simulink model "testmpc"  (R2021a)
settings: Solver=VariableStepAuto  StartTime=0.0  StopTime=10.0  RelTol=1e-3
undefined symbols (not defined in the file or in its folder): sigbuilder_block
libraries: mpclib x1
settings Model: Creator=uddin  LastModifiedBy=uddin

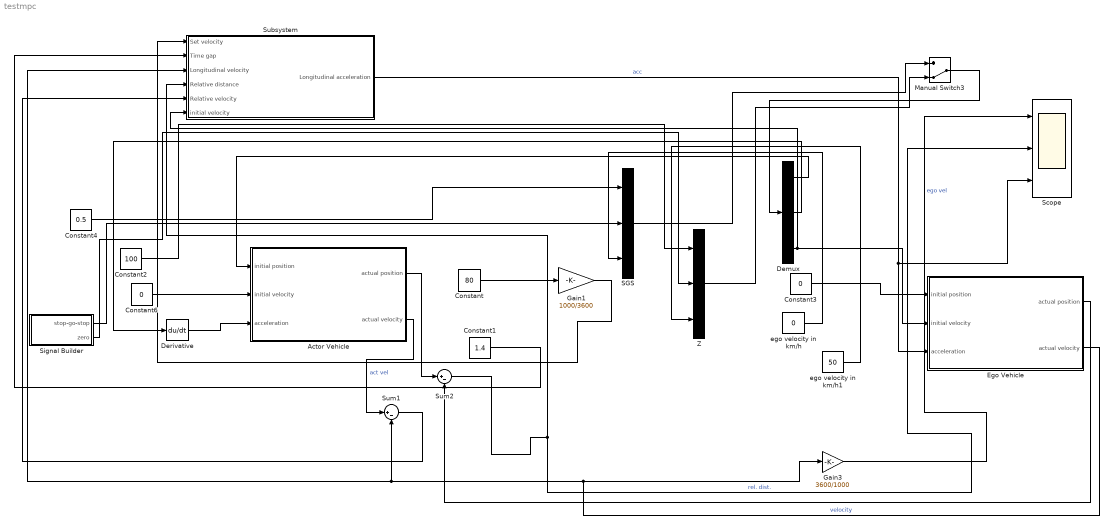
== system testmpc ==
  Actor Vehicle : Subsystem
  Constant : Constant  Value=80  SampleTime=1
  Constant1 : Constant  Value=1.4  SampleTime=1
  Constant2 : Constant  Value=100  SampleTime=1
  Constant3 : Constant  Value=0  SampleTime=1
  Constant4 : Constant  Value=0.5  SampleTime=1
  Constant6 : Constant  Value=0  SampleTime=1
  Demux : Demux  Outputs=3
  Derivative : Derivative
  Ego Vehicle : Subsystem
  Gain1 : Gain  Gain=1000/3600
  Gain3 : Gain  Gain=3600/1000
  Manual Switch3 : ManualSwitch  CurrentSetting=0
  SGS : Mux  Inputs=3
  Scope : Scope  NumInputPorts=3
  Signal Builder : Subsystem  Tag=STV Subsys  LoadFcn=sigbuilder_block('load');  StartFcn=sigbuilder_block('start');  StopFcn=sigbuilder_block('stop');  ClipboardFcn=sigbuilder_block('clipboard');  mask(Sigbuilder block){tuvar=[0:10]}
      mask help: Simulink:masks:SigbuilderBlock_MD
      mask init:
      | if ~strcmp(get_param(bdroot(gcbh),'SimulationStatus'),'stopped') tuvar = sigbuilder_block('maskInit'); end
      settings: CopyFcn=sigbuilder_block('copy');  DeleteFcn=sigbuilder_block('delete');  ModelCloseFcn=sigbuilder_block('modelClose');  PreSaveFcn=sigbuilder_block('preSave');  PauseFcn=sigbuilder_block('pause');  ContinueFcn=sigbuilder_block('continue');  NameChangeFcn=sigbuilder_block('namechange');  OpenFcn=sigbuilder_block('open',[393 134.4 550.8 400.2 ]);  CloseFcn=sigbuilder_block('close');
      mask Display: plot(0, 0, 100, 100,[2, 2, 32, 32, 2], [68, 8, 8, 68, 68],[32, 2], [38, 38], [32, 19, 2],[53, 60, 44], [32, 17, 17, 2],[16, 16, 31, 31]);txt = getActiveGroup(gcbh);text(2, 100, txt,'verticalAlignment', 'top');
  Subsystem : Subsystem
  Sum1 : Sum  Inputs=|+-
  Sum2 : Sum  Inputs=|+-
  Z : Mux  Inputs=3
  ego velocity in km/h : Constant  Value=0  SampleTime=1
  ego velocity in km/h1 : Constant  Value=50  SampleTime=1
  wires:
  Z/1 -> Manual Switch3/2
  Subsystem/1(Longitudinal acceleration) -> Ego Vehicle/3(acceleration), Scope/3  "acc"
  Demux/3 -> Subsystem/6(initial velocity), Ego Vehicle/2(initial velocity)
  Ego Vehicle/1(actual position) -> Sum2/2
  Constant1/1 -> Subsystem/2(Time gap)
  Sum1/1 -> Subsystem/5(Relative velocity)
  Gain3/1 -> Scope/1  "ego vel"
  Sum2/1 -> Subsystem/4(Relative distance), Scope/2  "rel. dist."
  Constant6/1 -> Actor Vehicle/2(initial velocity)
  Manual Switch3/1 -> Demux/1
  SGS/1 -> Manual Switch3/1
  Actor Vehicle/1(actual position) -> Sum2/1
  Constant4/1 -> SGS/1
  Derivative/1 -> Actor Vehicle/3(acceleration)
  ego velocity in km/h1/1 -> Z/3
  ego velocity in km/h/1 -> SGS/3
  Constant/1 -> Gain1/1
  Demux/1 -> Actor Vehicle/1(initial position)
  Actor Vehicle/2(actual velocity) -> Sum1/1  "act vel"
  Constant2/1 -> Z/1
  Ego Vehicle/2(actual velocity) -> Sum1/2, Subsystem/3(Longitudinal velocity), Gain3/1  "velocity"
  Signal Builder/2(zero) -> Z/2
  Demux/2 -> Derivative/1
  Gain1/1 -> Subsystem/1(Set velocity)
  Constant3/1 -> Ego Vehicle/1(initial position)
  Signal Builder/1(stop-go-stop) -> SGS/2

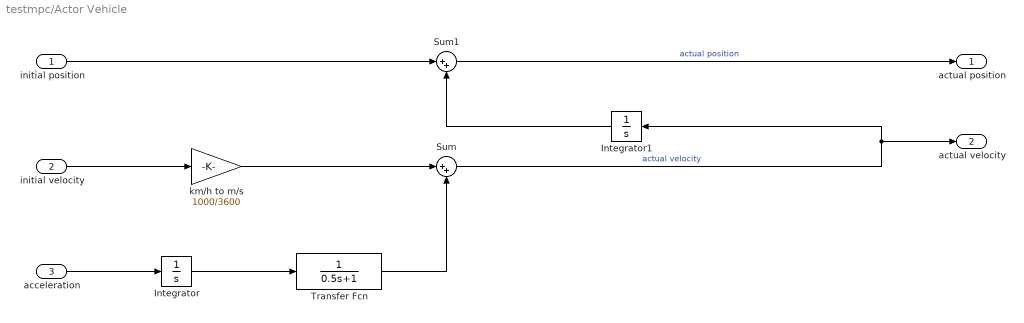
== system testmpc/Actor Vehicle ==
  initial position : Inport
  initial velocity : Inport  Port=2
  acceleration : Inport  Port=3
  Integrator : Integrator  ZeroCross=off
  Integrator1 : Integrator  ZeroCross=off
  Sum : Sum  Inputs=|++
  Sum1 : Sum  Inputs=|++
  Transfer Fcn : TransferFcn  Denominator=[0.5 1]
  km/h to m/s : Gain  Gain=1000/3600
  actual position : Outport
  actual velocity : Outport  Port=2
  wires:
  Integrator1/1 -> Sum1/2
  initial position/1 -> Sum1/1
  acceleration/1 -> Integrator/1
  Sum/1 -> Integrator1/1, actual velocity/1  "actual velocity"
  Sum1/1 -> actual position/1  "actual position"
  Integrator/1 -> Transfer Fcn/1
  Transfer Fcn/1 -> Sum/2
  initial velocity/1 -> km/h to m/s/1
  km/h to m/s/1 -> Sum/1

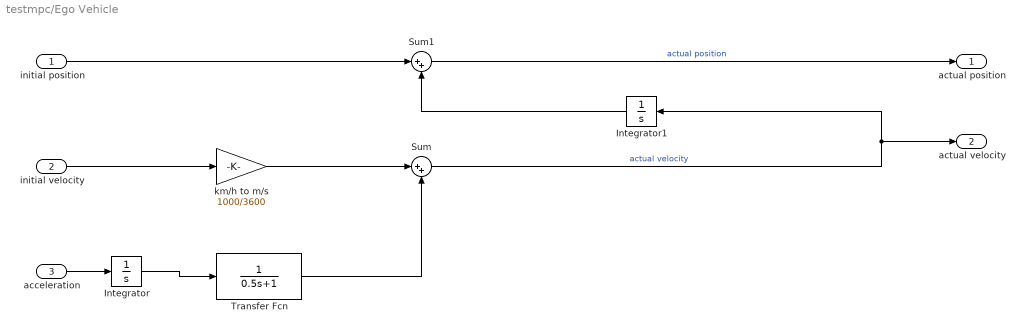
== system testmpc/Ego Vehicle ==
  initial position : Inport
  initial velocity : Inport  Port=2
  acceleration : Inport  Port=3
  Integrator : Integrator  ZeroCross=off
  Integrator1 : Integrator  ZeroCross=off
  Sum : Sum  Inputs=|++
  Sum1 : Sum  Inputs=|++
  Transfer Fcn : TransferFcn  Denominator=[0.5 1]
  km/h to m/s : Gain  Gain=1000/3600
  actual position : Outport
  actual velocity : Outport  Port=2
  wires:
  Sum1/1 -> actual position/1  "actual position"
  Sum/1 -> actual velocity/1, Integrator1/1  "actual velocity"
  acceleration/1 -> Integrator/1
  initial position/1 -> Sum1/1
  Integrator1/1 -> Sum1/2
  Integrator/1 -> Transfer Fcn/1
  Transfer Fcn/1 -> Sum/2
  initial velocity/1 -> km/h to m/s/1
  km/h to m/s/1 -> Sum/1

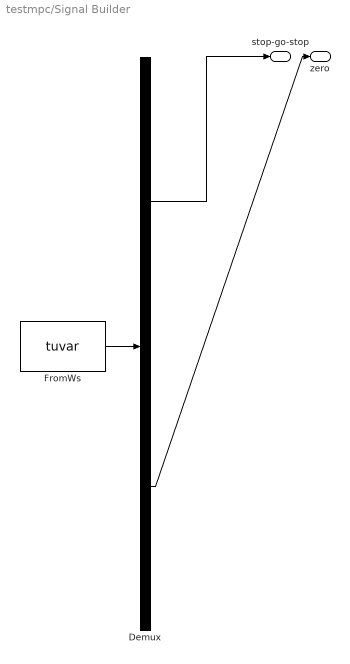
== system testmpc/Signal Builder ==
  Demux : Demux  Tag=STV Demux  Outputs=2
      settings: DisplayOption=none
  FromWs : FromWorkspace  Tag=STV FromWs  VariableName=tuvar
      SigBuilderData=|
      | common.afterFinalStr = 'Extrapolate'
      | common.sampleTime = 0
      | dataSet.timeRange = [0 30]
      | dataSet.name = 'Group 1'
      | sbobj.Groups.Name = 'Group 1'
      | sbobj.Groups.Signals(1).Name = 'stop-go-stop'
      | sbobj.Groups.Signals(1).XData = [0 5 10 20 25 30]
      | sbobj.Groups.Signals(1).YData = [0 0 2 2 0 0]
      | sbobj.Groups.Signals(2).Name = 'zero'
      | sbobj.Groups.Signals(2).XData = [0 30]
      | sbobj.Groups.Signals(2).YData = [0 0]
      | sbobj.Groups.TimeRange = [0 30]
  stop-go-stop : Outport  Tag=STV Outport
  zero : Outport  Tag=STV Outport  Port=2
  wires:
  FromWs/1 -> Demux/1
  Demux/1 -> stop-go-stop/1
  Demux/2 -> zero/1

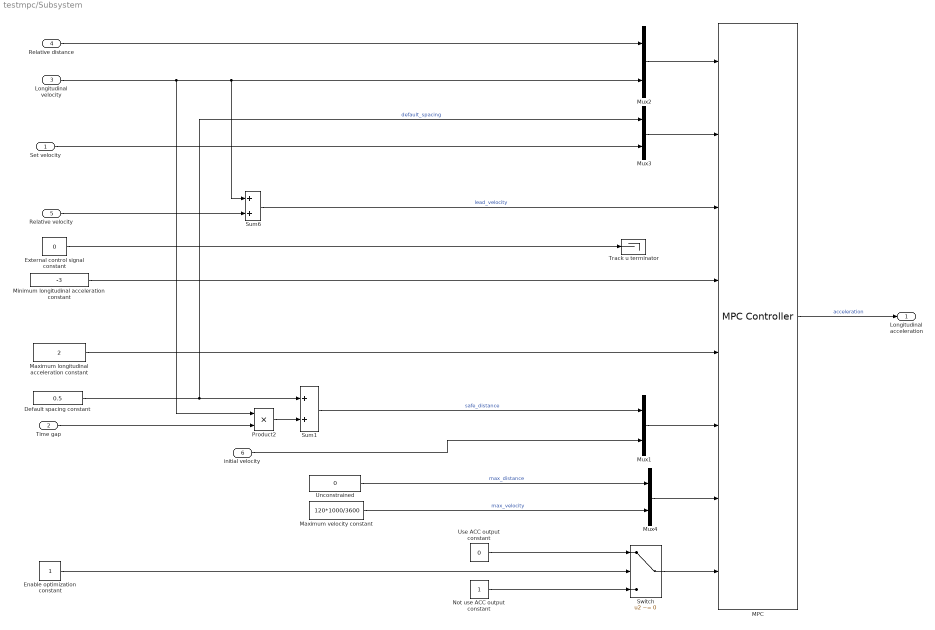
== system testmpc/Subsystem ==
  Set velocity : Inport
  Time gap : Inport  Port=2
  Longitudinal velocity : Inport  Port=3
  Relative distance : Inport  Port=4
  Relative velocity : Inport  Port=5
  initial velocity : Inport  Port=6
  Default spacing constant : Constant  Value=0.5  OutDataTypeStr=DataType
  Enable optimization constant : Constant  OutDataTypeStr=double
  External control signal constant : Constant  Value=0  OutDataTypeStr=double
  MPC : mpclib/MPC Controller  SCDEnableBlockLinearizationSpecification=on  mpcobj=mpcobj  is_multiple=0  enable_value=0  return_u0=off  updateMPCinCallerWorkspace=off  md_inport=on  mv_inport=off  uref_inport=off  return_cost=off  return_mvseq=off  return_qpstatus=off  return_xseq=off  return_state=off  return_ovseq=off  state_inport=off  umin_inport=on  umax_inport=on  ymin_inport=on  ymax_inport=on  cc_inport=off  ywt_inport=off  uwt_inport=off  duwt_inport=off  rhoeps_inport=off  pm_inport=off  MaximumP=10  HorizonChoice=FixedHorizon  n_ts=0.5  n_p=15  n_mv=1  n_md=1  n_ud=0  n_mo=2  n_uo=0  BlockDataType=double  SampleTimeInherited=off  switch_inport=on
  Maximum longitudinal acceleration constant : Constant  Value=2  OutDataTypeStr=double
  Maximum velocity constant : Constant  Value=120*1000/3600  OutDataTypeStr=DataType
  Minimum longitudinal acceleration constant : Constant  Value=-3  OutDataTypeStr=double
  Mux{1..4} (4 alike) : Mux  Inputs=[1 1]
  Not use ACC output constant : Constant  OutDataTypeStr=DataType
  Product2 : Product
  Sum1 : Sum
  Sum6 : Sum
  Switch : Switch  Criteria=u2 ~= 0
  Track u terminator : Terminator
  Unconstrained : Constant  Value=0  OutDataTypeStr=DataType
  Use ACC output constant : Constant  Value=0  OutDataTypeStr=DataType
  Longitudinal acceleration : Outport  PortDimensions=1  VectorParamsAs1DForOutWhenUnconnected=off
  wires:
  Longitudinal velocity/1 -> Mux2/2, Sum6/1, Product2/1
  Default spacing constant/1 -> Mux3/1, Sum1/1  "default_spacing"
  Enable optimization constant/1 -> Switch/2
  Use ACC output constant/1 -> Switch/1
  Relative velocity/1 -> Sum6/2
  Mux2/1 -> MPC/1
  Maximum longitudinal acceleration constant/1 -> MPC/5
  Mux3/1 -> MPC/2
  Switch/1 -> MPC/8
  Mux1/1 -> MPC/6
  Mux4/1 -> MPC/7
  Time gap/1 -> Product2/2
  Product2/1 -> Sum1/2
  Maximum velocity constant/1 -> Mux4/2  "max_velocity"
  Not use ACC output constant/1 -> Switch/3
  Minimum longitudinal acceleration constant/1 -> MPC/4
  MPC/1 -> Longitudinal acceleration/1  "acceleration"
  External control signal constant/1 -> Track u terminator/1
  Unconstrained/1 -> Mux4/1  "max_distance"
  Sum6/1 -> MPC/3  "lead_velocity"
  Relative distance/1 -> Mux2/1
  Sum1/1 -> Mux1/1  "safe_distance"
  Set velocity/1 -> Mux3/2
  initial velocity/1 -> Mux1/2
